simulink model "BalancingMotorCycle"  (R2023b)
settings: Solver=FixedStepAuto  StartTime=0.0  StopTime=inf  RelTol=1e-3  EnableMultiTasking=on
model workspace (MAT data in the model file):
  Ts = Simulink.Parameter
  Ts.Value = 0.01
  Ts.DataType = 'auto'
  Ts.Complexity = 'real'
  Ts.Dimensions = [1 1]
libraries: arduinomotorcarrierlib x2, mkrmotorcarrierlib x2, simulink x1, eeGeneralControl x1, arduinosensorlib x1
settings Model: ExtModeTrigDuration=2  Creator=bkhusain  LastModifiedBy=anura
settings SolverCC: AlgebraicLoopSolver=TrustRegion
settings OptimizationCC: EnhancedBackFolding=on  PassReuseOutputArgsThreshold=0  MaxStackSize=64  OptimizeBlockOrder=speed  DifferentSizesBufferReuse=on
settings DebuggingCC: MultiTaskRateTransMsg=warning  ParameterTunabilityLossMsg=error  UnconnectedInputMsg=warning  UnconnectedOutputMsg=warning  UnconnectedLineMsg=warning
settings HardwareCC: ProdBitPerPointer=32  ProdBitPerSizeT=32  ProdBitPerPtrDiffT=32  ProdLargestAtomicInteger=Long  ProdLargestAtomicFloat=Double  ProdWordSize=32  ProdHWDeviceType=ARM Compatible->ARM Cortex  UseEmbeddedCoderFeatures=off  UseSimulinkCoderFeatures=off
settings ModelReferenceCC: EnableRefExpFcnMdlSchedulingChecks=on
settings SFSimCC: MATLABDynamicMemAlloc=off
settings RTWCC: Description=Embedded Coder  SystemTargetFile=ert.tlc  HardwareBoard=Arduino Nano 33 IoT  TemplateMakefile=ert_default_tmf  Toolchain=Arduino ARM  BuildConfiguration=Faster Runs
settings CodeAppCC: ForceParamTrailComments=on  OperatorAnnotations=on
settings ERTTargetCC: ERTCustomFileBanners=off  SupportContinuousTime=on  SupportNonInlinedSFcns=on  RemoveResetFunc=off  SupportVariableSizeSignals=on  ModelStepFunctionPrototypeControlCompliant=off  ExtModeStaticAllocSize=8192

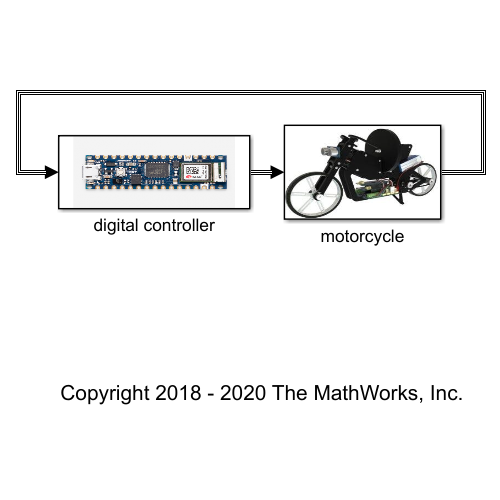
[thumbnail: Simulink's stored preview of the top-level diagram]
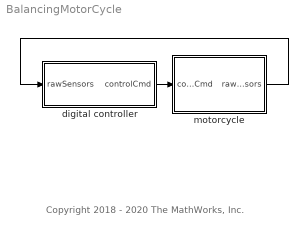
== system BalancingMotorCycle ==
  note: Copyright 2018 - 2020 The MathWorks, Inc.
  digital controller : Subsystem
      mask Display: image('$imagefile'); % Use "Edit Image" on toolstrip to change.
  motorcycle : Subsystem
      mask Display: image('$imagefile'); % Use "Edit Image" on toolstrip to change.
  wires:
  digital controller/1(controlCmd) -> motorcycle/1(controlCmd)
  motorcycle/1(rawSensors) -> digital controller/1(rawSensors)

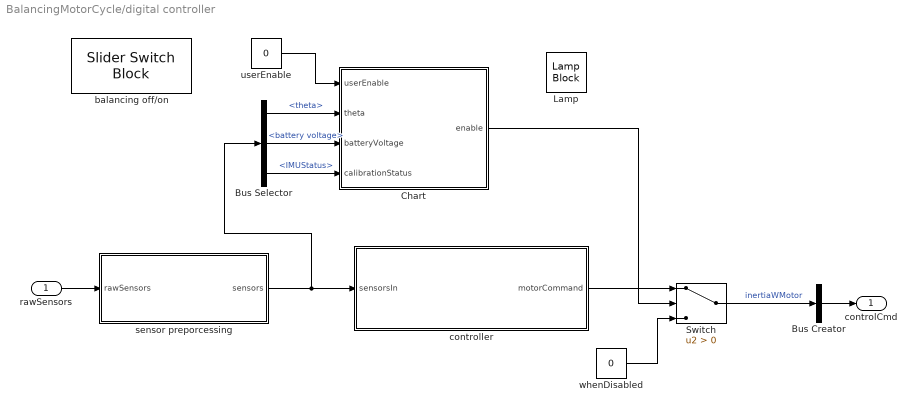
== system BalancingMotorCycle/digital controller ==
  rawSensors : Inport
  Bus Creator : BusCreator  Inputs=1
  Bus Selector : BusSelector  OutputSignals=theta,battery voltage,IMUStatus
  Chart : Stateflow chart  TreatAsAtomicUnit=on
  Lamp : LampBlock
  Switch : Switch  Criteria=u2 > Threshold  SaturateOnIntegerOverflow=off  InputSameDT=off
  balancing off/on : SliderSwitchBlock  LabelPosition=Hide
      settings: Values={{'Off', 'On'}, [0 1]}
  controller : Subsystem
  sensor preporcessing : Subsystem
  userEnable : Constant  Value=0  SampleTime=Ts
  whenDisabled : Constant  Value=0  SampleTime=Ts
  controlCmd : Outport
  wires:
  Switch/1 -> Bus Creator/1  "inertiaWMotor"
  Bus Creator/1 -> controlCmd/1
  rawSensors/1 -> sensor preporcessing/1(rawSensors)
  sensor preporcessing/1(sensors) -> controller/1(sensorsIn), Bus Selector/1
  whenDisabled/1 -> Switch/3
  Chart/1(enable) -> Switch/2
  Bus Selector/1 -> Chart/2(theta)  "<theta>"
  Bus Selector/2 -> Chart/3(batteryVoltage)  "<battery voltage>"
  Bus Selector/3 -> Chart/4(calibrationStatus)  "<IMUStatus>"
  userEnable/1 -> Chart/1(userEnable)
  controller/1(motorCommand) -> Switch/1

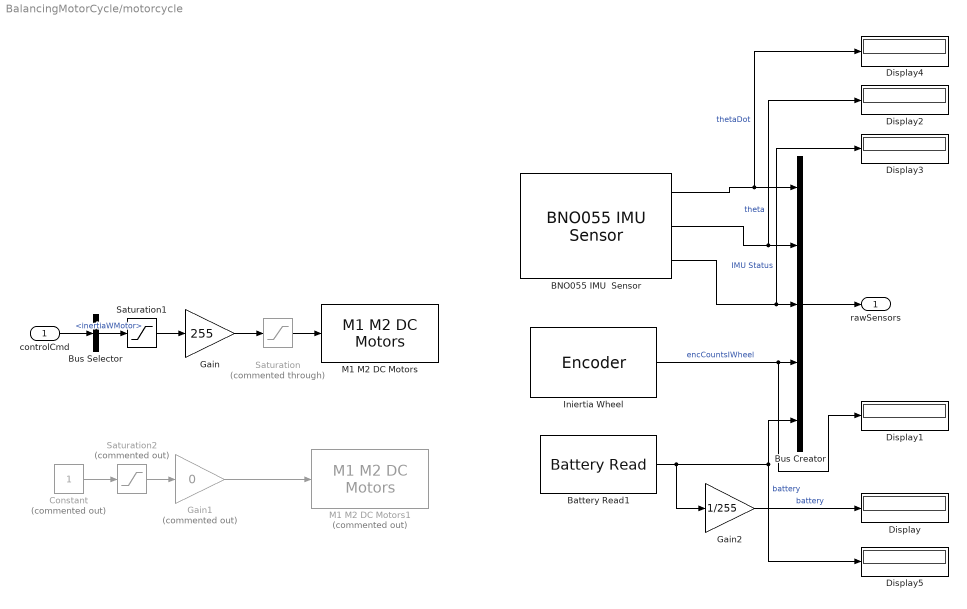
== system BalancingMotorCycle/motorcycle ==
  controlCmd : Inport
  BNO055 IMU  Sensor : arduinosensorlib/BNO055 IMU Sensor  SlaveAddress=0x28  OperationMode=Fusion  Accel=off  AngularRate=on  MagField=off  EulerAngles=on  Quat=off  LinearAccel=off  GravityVector=off  Status=on  Timestamp=off  AccelRange=4G  AccelBW=62.5 Hz  GyroRange=2000 dps  GyroBW=32 Hz  MagODR=10 Hz  spf=1  SampleTime=Ts  blockPlatform=ARDUINO  QueueSizeFactor=1
  Battery Read1 : arduinomotorcarrierlib/Battery Read  SlaveAddress=uint8( hex2dec( '66' ) )  blockPlatform=ARDUINO  SampleTime=0.1
  Bus Creator : BusCreator  Inputs=5
  Bus Selector : BusSelector  OutputSignals=inertiaWMotor
  Constant : Constant  Commented=on
  Display{,1..5} (6 alike) : Display
  Gain : Gain  Gain=255
  Gain1 : Gain  Commented=on  Gain=0
  Gain2 : Gain  Gain=1/255
  Iniertia Wheel : arduinomotorcarrierlib/Encoder  SlaveAddress=uint8( hex2dec( '66' ) )  blockPlatform=ARDUINO  Encoder=1  ShowSpeed=off  ResetOption=on  SampleTime=Ts
  M1 M2 DC Motors : mkrmotorcarrierlib/M1 M2 DC Motors  SlaveAddress=uint8( hex2dec( '66' ) )  blockPlatform=ARDUINO  MotorNumber=M1  MotorCarrierPWMFreq=100
  M1 M2 DC Motors1 : mkrmotorcarrierlib/M1 M2 DC Motors  Commented=on  SlaveAddress=uint8( hex2dec( '66' ) )  blockPlatform=ARDUINO  MotorNumber=M2  MotorCarrierPWMFreq=100
  Saturation : Saturate  Commented=through  UpperLimit=255  LowerLimit=-255
  Saturation1 : Saturate  UpperLimit=50  LowerLimit=-50
  Saturation2 : Saturate  Commented=on  UpperLimit=255  LowerLimit=-255
  rawSensors : Outport
  wires:
  BNO055 IMU  Sensor/1 -> Display4/1, Bus Creator/1  "thetaDot"
  BNO055 IMU  Sensor/2 -> Display2/1, Bus Creator/2  "theta"
  BNO055 IMU  Sensor/3 -> Display3/1, Bus Creator/3  "IMU Status"
  Iniertia Wheel/1 -> Display1/1, Bus Creator/4  "encCountsIWheel"
  Battery Read1/1 -> Bus Creator/5, Display5/1, Gain2/1  "battery"
  Bus Creator/1 -> rawSensors/1
  controlCmd/1 -> Bus Selector/1
  Gain/1 -> Saturation/1
  Bus Selector/1 -> Saturation1/1  "<inertiaWMotor>"
  Saturation/1 -> M1 M2 DC Motors/1
  Gain2/1 -> Display/1  "battery"
  Gain1/1 -> M1 M2 DC Motors1/1
  Constant/1 -> Saturation2/1
  Saturation2/1 -> Gain1/1
  Saturation1/1 -> Gain/1

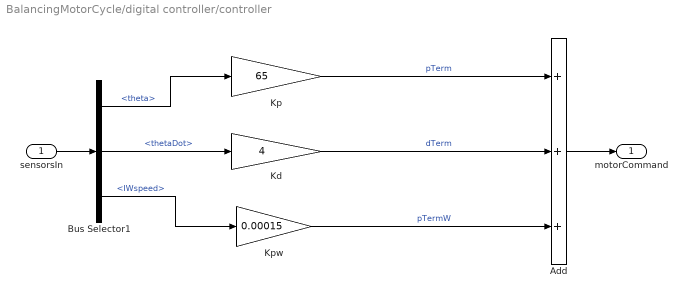
== system BalancingMotorCycle/digital controller/controller ==
  sensorsIn : Inport
  Add : Sum  Inputs=+++
  Bus Selector1 : BusSelector  OutputSignals=theta,thetaDot,IWspeed
  Kd : Gain  Gain=4
  Kp : Gain  Gain=65
  Kpw : Gain  Gain=0.00015
  motorCommand : Outport
  wires:
  Bus Selector1/3 -> Kpw/1  "<IWspeed>"
  Kpw/1 -> Add/3  "pTermW"
  Bus Selector1/2 -> Kd/1  "<thetaDot>"
  Bus Selector1/1 -> Kp/1  "<theta>"
  sensorsIn/1 -> Bus Selector1/1
  Add/1 -> motorCommand/1
  Kp/1 -> Add/1  "pTerm"
  Kd/1 -> Add/2  "dTerm"

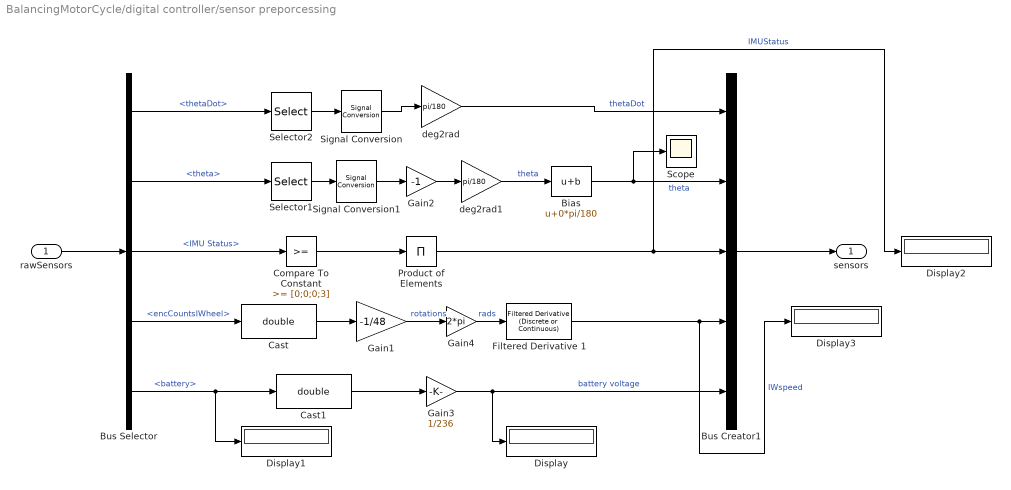
== system BalancingMotorCycle/digital controller/sensor preporcessing ==
  rawSensors : Inport
  Bias : Bias  Bias=0*pi/180  SaturateOnIntegerOverflow=off
  Bus Creator1 : BusCreator  Inputs=5
  Bus Selector : BusSelector  OutputSignals=thetaDot,theta,IMU Status,encCountsIWheel,battery
  Cast : DataTypeConversion  OutDataTypeStr=double  SaturateOnIntegerOverflow=off  RndMeth=Floor
  Cast1 : DataTypeConversion  OutDataTypeStr=double  SaturateOnIntegerOverflow=off  RndMeth=Floor
  Compare To Constant : simulink/Logic and Bit Operations/Compare To Constant  relop=>=  const=[0;0;0;3]  OutDataTypeStr=boolean
  Display{,1..3} (4 alike) : Display
  Filtered Derivative 1 : eeGeneralControl/Filtered Derivative (Discrete or Continuous)  K=1  T=0.1  B=inf  A=-inf  minRatio=10  init_option=Inherited from block input  x0=0  Ts=Ts
  Gain1 : Gain  Gain=-1/48
  Gain2 : Gain  Gain=-1
  Gain3 : Gain  Gain=1/236
  Gain4 : Gain  Gain=2*pi
  Product of Elements : Product  Inputs=*
  Scope : Scope
  Selector1 : Selector  InputPortWidth=3  IndexOptions=Index vector (dialog)  Indices=[2]  OutputSizes=1
  Selector2 : Selector  InputPortWidth=3  IndexOptions=Index vector (dialog)  Indices=[2]  OutputSizes=1
  Signal Conversion : SignalConversion  OverrideOpt=off
  Signal Conversion1 : SignalConversion  OverrideOpt=off
  deg2rad : Gain  Gain=pi/180
  deg2rad1 : Gain  Gain=pi/180
  sensors : Outport
  wires:
  Bus Selector/4 -> Cast/1  "<encCountsIWheel>"
  Compare To Constant/1 -> Product of Elements/1
  Bus Selector/5 -> Display1/1, Cast1/1  "<battery>"
  Selector2/1 -> Signal Conversion/1
  Bus Selector/2 -> Selector1/1  "<theta>"
  Selector1/1 -> Signal Conversion1/1
  Cast1/1 -> Gain3/1
  Bus Selector/3 -> Compare To Constant/1  "<IMU Status>"
  rawSensors/1 -> Bus Selector/1
  Product of Elements/1 -> Display2/1, Bus Creator1/3  "IMUStatus"
  Filtered Derivative 1/1 -> Display3/1, Bus Creator1/4  "IWspeed"
  deg2rad1/1 -> Bias/1  "theta"
  Bus Selector/1 -> Selector2/1  "<thetaDot>"
  Gain3/1 -> Display/1, Bus Creator1/5  "battery voltage"
  Bus Creator1/1 -> sensors/1
  Signal Conversion1/1 -> Gain2/1
  Gain2/1 -> deg2rad1/1
  Signal Conversion/1 -> deg2rad/1
  Cast/1 -> Gain1/1
  Gain1/1 -> Gain4/1  "rotations"
  Gain4/1 -> Filtered Derivative 1/1  "rads"
  deg2rad/1 -> Bus Creator1/1  "thetaDot"
  Bias/1 -> Scope/1, Bus Creator1/2  "theta"

== stateflow chart BalancingMotorCycle/digital controller/Chart ==
  state checkFallen [parallel]
    settings: executionOrder=1
    state fallen
      entry: upright = false
    state standing
      entry: upright = true
    (default) -> fallen
    fallen -> standing : [abs(theta) <pi*12/180]
    standing -> fallen : [abs(theta) > pi*12/180]
  state checkIMUCalib [parallel]
    settings: executionOrder=2
    state imuNotCalibrated
      entry:
      IMUCalibrated = false;
    state imuCalibrated
      entry:
      IMUCalibrated = true;
    (default) -> imuNotCalibrated
    imuNotCalibrated -> imuCalibrated : [calibrationStatus == true]
  state checkBattery [parallel]
    settings: executionOrder=3
    state batteryNotCharged
      entry:
      batteryOK = false;
    state batteryCharged
      entry:
      batteryOK = true;
    (default) -> batteryNotCharged
    batteryCharged -> batteryNotCharged : [batteryVoltage < 3.0]
    batteryNotCharged -> batteryCharged : [batteryVoltage >= 3.0]
  state calculateEnable [parallel]
    settings: executionOrder=4
    state disableControl
      entry: enable = false
    state enableControl
      entry: enable = true
    (default) -> disableControl
    disableControl -> enableControl : [userEnable&& batteryOK && IMUCalibrated && upright]
    enableControl -> disableControl : [not(userEnable) || not(batteryOK) || not(IMUCalibrated) || not(upright)]
  data: userEnable input; theta input; enable output; batteryVoltage input; calibrationStatus input; upright local; IMUCalibrated local; batteryOK local
